simulink model "CD1_CityDrain_Library_outdated"  (Simulink 5.0)
settings: Solver=FixedStepDiscrete  StartTime=0  StopTime=36000  FixedStep=300  RelTol=1e-3
settings Model: LastModifiedBy=c81523  TimeSaveName=cd_time  LimitDataPoints=off

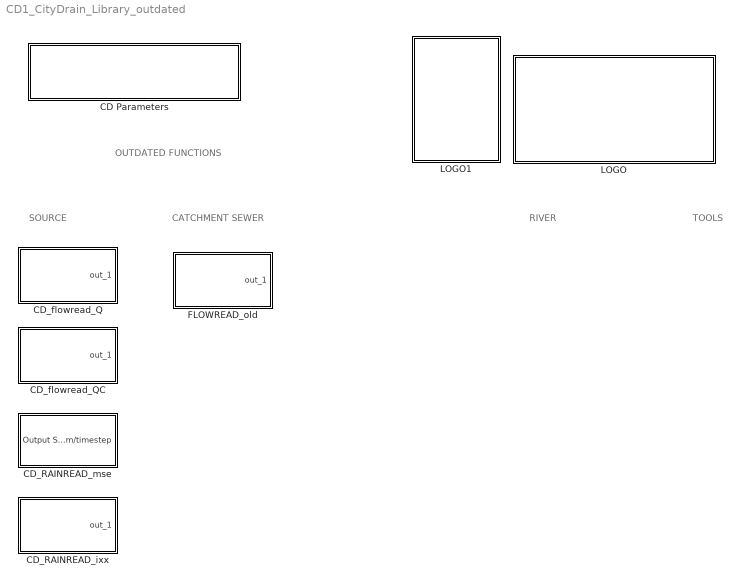
== system CD1_CityDrain_Library_outdated ==
  note: TOOLS
  note: SOURCE
  note: RIVER
  note: CATCHMENT
      | SEWER
  note: OUTDATED FUNCTIONS
  CD Parameters : Subsystem  mask(City Drain 1.0 - Simulation parameters ){t_step=300, t_start=0, t_stop=36000}
      mask prompts: t_step "Sampling Time [s]"; t_start "Start Time [s]"; t_stop "Stop Time [s]"
      mask help:
      | Block that sets the global parameters required in City Drain 1.0. Following paramters are set without user's input:
      |
      | - 'Solver' --> 'FixedStepDiscrete'
      | - 'TimeSaveName' --> 'cd_time'
      | - 'Decimation' --> '1'
      | - 'LimitDataPoints' -->  'off'
      mask init:
      | % toplevel systems' name --> Plant file name;
      | tls=bdroot(gcb); 
      | set_param(tls, 'Solver', 'FixedStepDiscrete'); 
      | set_param(tls, 'TimeSaveName', 'cd_time');
      | set_param(tls, 'Decimation', '1');
      | set_param(tls, 'LimitDataPoints', 'off');
      | set_param(tls, 'ScreenColor', 'white');
      | 
      | tstep_char=num2str(t_step); % Setting the discrete time step
      | set_param(tls, 'FixedStep', tstep_char); 
      | 
      | tstart_char=num2str(t_start); % Setting the start time
      | set_param(tls, 'StartTime', tstart_char); 
      | 
      | tstop_char=num2str(t_stop); % Setting the stop time
      | set_param(tls, 'StopTime', tstop_char);
      mask Display:
      | plot(0,0,100,100);
      | 
      | text(50,65,'CITY DRAIN','HorizontalAlignment','center');
      | text(50,35,'PARAMETERS','HorizontalAlignment','center');
      | 
      | 
      | image(imread('CityDrain_SimParam.jpg'))
  CD_RAINREAD_ixx : Subsystem  mask(Rain Read: ixx-format){file0='Rain_ixx_1980_2m_summer.ixx'}
      mask prompts: file0 "Inputfile"
      mask help:
      | Read raindata from ASCII File in ixx format.
      |
      | Timesteps in the data must match the simulation time steps !!
      |
      | Used function:
      | CD1_mfun_rainread_ixx.m
      mask init:
      | % reading the toplevel systems' name 
      | % --> Plant file name;
      | tls=bdroot(gcb); 
      | % Obtaining the fixed sampling time
      | t_samp_char=get_param(tls, 'FixedStep');
      | % Convertion to numeric value
      | t_sample = str2num(t_samp_char);
      mask Display:
      | plot(0,0,100,100);
      | text(35,75,'ixx-format');
      | text(60,40,'RAIN');
      | text(60,20,'READ');
      | 
      | plot(
      | [5 10 10 15 15 20 20 25 25 30 30 40 40 45],
      | [0 0 20 20 40 40 60 60 30 30 0 0 0 0]+20);
  CD_RAINREAD_mse : Subsystem  mask(RainRead: mse-format){filename='Rain_mse_1981.mse'}
      mask prompts: filename "File Name 'Raindata.mse'"
      mask help:
      | Reads rain data from the specified  file in mse - format (modified DHI Mouse format).
      | Precipitation given in [1000*mm/sec] is converted to discrete volumetric values in [mm/timestep]. Simulation is stopped with last recorded precipitation.
      |
      | Timesteps in the data must match the simulation time steps !!
      |
      | Required time steps for sampling are inherited from global setting.
      mask init:
      | % reading the toplevel systems' name 
      | % --> Plant file name;
      | tls=bdroot(gcb); 
      | % Obtaining the fixed sampling time
      | t_samp_char=get_param(tls, 'FixedStep');
      | % Convertion to numeric value
      | tstep = str2num(t_samp_char);
      mask Display:
      | plot(0,0,100,100);
      | text(35,75,'mse-format');
      | text(60,40,'RAIN');
      | text(60,20,'READ');
      | 
      | plot(
      | [5 10 10 15 15 20 20 25 25 30 30 40 40 45],
      | [0 0 20 20 40 40 60 60 30 30 0 0 0 0]+20);
  CD_flowread_Q : Subsystem  mask(CD1_mfun_flowread_Q.m){table0='Input_Flow_Q_01.txt'}
      mask prompts: table0 "File cotaining matrix of hydrograph"
      mask help:
      | Reads flowdata (Q) from ascii file.
      |
      | Timesteps in the data must match the simulation time steps !!
      |
      | Used function: CD1_mfun_flowread_Q.m
      mask init:
      | table=CD1_mfun_flowread_Q_old(table0); 
      | h=size(table);m=max(table(:,h(2)));
      | n=min(table(:,h(2)))/(m+eps);x=max(table(:,1));
      | z=1.643;
      | 
      | % reading the toplevel systems' name 
      | % --> Plant file name;
      | tls=bdroot(gcb); 
      | % Obtaining the fixed sampling time
      | t_samp_char=get_param(tls, 'FixedStep');
      | % Convertion to numeric value
      | t_sample = str2num(t_samp_char);
      mask Display: plot(-x/z*0.1,(n-0.2)*m,x+x/z*0.1,m+m/10,table(:,1),table(:,h(2)),x/z*[-0.1,0.05],[n*m,(n-0.2)*m])
  CD_flowread_QC : Subsystem  mask( CD1_mfun_flowread_QC){table0='Input_Flow_QC_01.txt', n_comp=1}
      mask prompts: table0 "Filename"; n_comp "Number of pollutants n"
      mask help:
      | Reads flowdata (Q) and substance concentration (Ci) associated from ascii file.
      |
      | Timesteps in the data must match the simulation time steps !!
      |
      | Used function: CD1_mfun_flowread_QC.m
      mask init:
      | table=CD1_mfun_flowread_QC_old(table0,n_comp);
      | 
      | h=size(table);m=max(table(:,h(2)));
      | n=min(table(:,h(2)))/(m+eps);x=max(table(:,1));
      | z=1.643;
      | 
      | % reading the toplevel systems' name 
      | % --> Plant file name;
      | tls=bdroot(gcb); 
      | % Obtaining the fixed sampling time
      | t_samp_char=get_param(tls, 'FixedStep');
      | % Convertion to numeric value
      | t_sample = str2num(t_samp_char);
      mask Display:
      | plot(0,0,100,100);
      | 
      | text(20,30,'Flowread');
      | 
      | text(20,10,'Q and C');
      | 
      | 
      | plot(
      | [5 20 20 30 30 40 40 50 50 60 60 70 70 70],
      | [0 0 10 10 20 20 40 40 20 20 0 0 0 0]+60);
      | plot(
      | [5 20 20 30 30 40 40 50 50 60 60 70 70 70],
      | [0 0 10 10 20 20 30 30 10 10 0 0 0 0]+40);
  FLOWREAD_old : Subsystem  mask(CD1_flowread){table0='Input_CSO_QC_Test_3.txt', dtype=Grab sample, crep=on}
      mask prompts: table0 "Filename"; dtype "Data type"; crep "Cylic repitation"
      mask help:
      | Reads flowdata (Q) and substance concentration (Ci) associated from ascii file.
      |
      | Used function: CD1_sfun_flowread.m
      mask init:
      | table=CD1_mfun_flowread(table0);
      | 
      | 
      | % reading the toplevel systems' name 
      | % --> Plant file name;
      | tls=bdroot(gcb); 
      | % Obtaining the fixed sampling time
      | t_samp_char=get_param(tls, 'FixedStep');
      | % Convertion to numeric value
      | tstep = str2num(t_samp_char);
      mask StyleString: edit,popup(Composite sample|Grab sample),checkbox
      mask Display:
      | plot(0,0,100,100);
      | 
      | text(50,20,'FLOWREAD_old','HorizontalAlignment','center');
      | 
      | plot(
      | [5 10 10 15 15 20 20 25 25 30 30 35 35 40],
      | [0 0 10 10 20 20 40 40 20 20 0 0 0 0]+50);
      | plot(
      | [5 10 15 20 25 30 35 ]+50,
      | [0 5 10 15 30 20 0]+50);
  LOGO : Subsystem
      mask Type: LOGO CITY DRAIN
      mask Description:
      | Displays the City Drain Logo in Color
      | 
      | Source file:
      | City Drain Logo_c_small.tif
      mask Help:
      | Displays the City Drain Logo in Color
      | 
      | Source file:
      | City Drain Logo_c_small.tif
      mask Display:
      | image(imread('CityDrainLogo_C1.jpg'));
      | text(10,50,'CITY DRAIN 1.0','HorizontalAlignment','left');
      | text(10,20,'Logo could not be displayed','HorizontalAlignment','left');
  LOGO1 : Subsystem
      mask Type: LOGO CITY DRAIN
      mask Description:
      | Displays the City Drain Logo in Color
      | 
      | Source file:
      | CityDrainLogo_C1.jpg
      mask Display:
      | image(imread('LOGO_IUT4C.jpg'));
      | text(10,50,'IUT, University of Innsbruck','HorizontalAlignment','left');
      | text(10,20,'Logo could not be displayed','HorizontalAlignment','left');

== system CD1_CityDrain_Library_outdated/CD Parameters ==

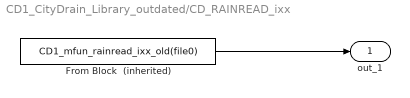
== system CD1_CityDrain_Library_outdated/CD_RAINREAD_ixx ==
  From Block  (inherited) : FromWorkspace  VariableName=CD1_mfun_rainread_ixx_old(file0)  SampleTime=t_sample  OutputAfterFinalValue=Setting to zero
  out_1 : Outport
  wires:
  From Block  (inherited)/1 -> out_1/1

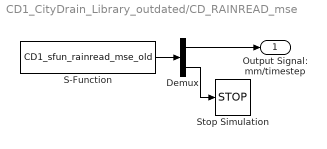
== system CD1_CityDrain_Library_outdated/CD_RAINREAD_mse ==
  Demux : Demux  Outputs=2
  S-Function : S-Function  FunctionName=CD1_sfun_rainread_mse_old  Parameters=filename,tstep
  Stop Simulation : Stop
  Output Signal: mm/timestep : Outport
  wires:
  Demux/1 -> Output Signal: mm/timestep/1
  Demux/2 -> Stop Simulation/1
  S-Function/1 -> Demux/1

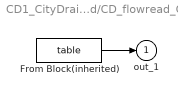
== system CD1_CityDrain_Library_outdated/CD_flowread_Q ==
  From Block(inherited) : FromWorkspace  VariableName=table  SampleTime=t_sample  Interpolate=off  OutputAfterFinalValue=Setting to zero
  out_1 : Outport
  wires:
  From Block(inherited)/1 -> out_1/1

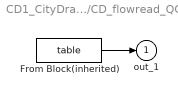
== system CD1_CityDrain_Library_outdated/CD_flowread_QC ==
  From Block(inherited) : FromWorkspace  VariableName=table  SampleTime=t_sample  Interpolate=off  OutputAfterFinalValue=Setting to zero
  out_1 : Outport
  wires:
  From Block(inherited)/1 -> out_1/1

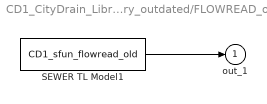
== system CD1_CityDrain_Library_outdated/FLOWREAD_old ==
  SEWER TL Model1 : S-Function  FunctionName=CD1_sfun_flowread_old  Parameters=dtype,crep,table,tstep
  out_1 : Outport
  wires:
  SEWER TL Model1/1 -> out_1/1

== system CD1_CityDrain_Library_outdated/LOGO ==

== system CD1_CityDrain_Library_outdated/LOGO1 ==
